simulink model "cte1"  (R2024b)
settings: Solver=ode15s  StartTime=0.0  StopTime=10.0  MaxStep=0.001  RelTol=1e-5
libraries: fl_lib x14, nesl_utility x6
settings Model: Creator=Apeksha  LastModifiedBy=hp

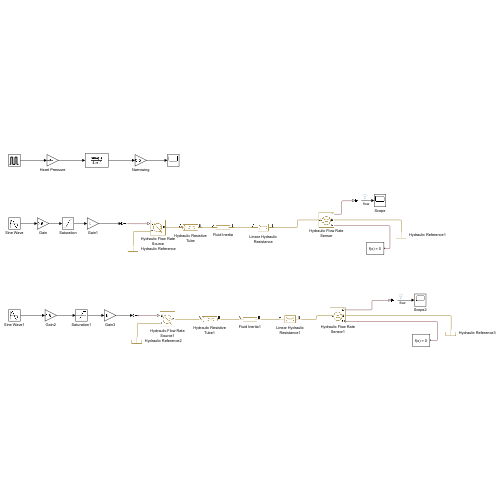
[thumbnail: Simulink's stored preview of the top-level diagram]
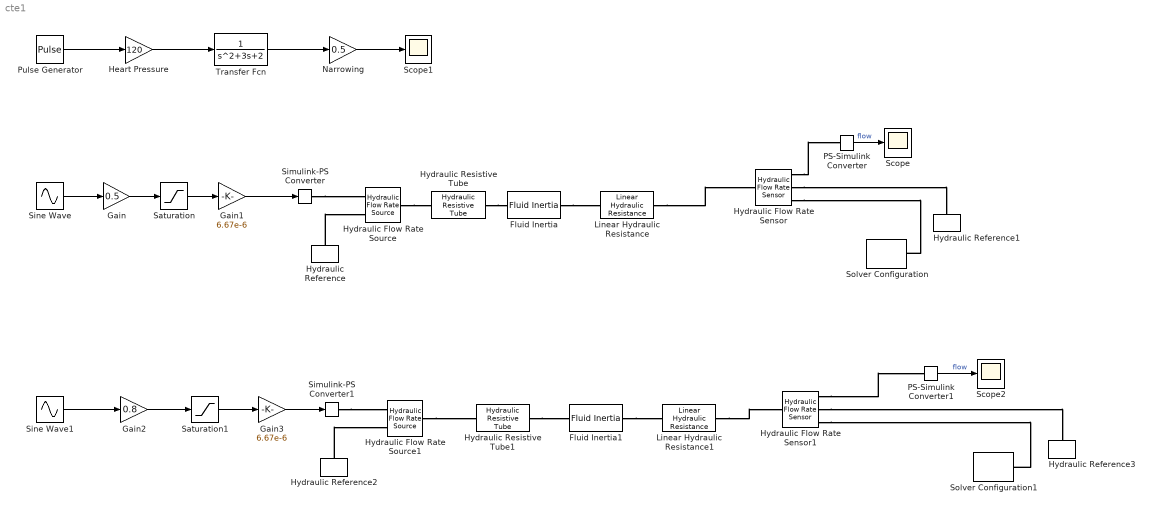
== system cte1 ==
  Fluid Inertia : fl_lib/Hydraulic/Hydraulic Elements/Fluid Inertia  area=0.8e-4 m^2  length=1 m  q_specify=on  q_priority=High  q=0 m^3/s  q_nominal_specify=off  q_nominal_value=1  q_nominal_unit=m^3/s  p_specify=on  p_priority=None  p=0 Pa  p_nominal_specify=off  p_nominal_value=1  p_nominal_unit=Pa
      settings: InternalSimscapePortConfiguration="{\"Bottom\":[],\"Left\":[{\"id\":\"A\",\"label\":\"A\",\"type\":\"foundation.hydraulic.hydraulic\"}],\"Right\":[{\"id\":\"B\",\"label\":\"B\",\"type\":\"foundation.hydraulic.hydraulic\"}],\"Top\":[]}"
  Fluid Inertia1 : fl_lib/Hydraulic/Hydraulic Elements/Fluid Inertia  area=0.8e-4 m^2  length=1 m  q_specify=on  q_priority=High  q=0 m^3/s  q_nominal_specify=off  q_nominal_value=1  q_nominal_unit=m^3/s  p_specify=on  p_priority=None  p=0 Pa  p_nominal_specify=off  p_nominal_value=1  p_nominal_unit=Pa
      settings: InternalSimscapePortConfiguration="{\"Bottom\":[],\"Left\":[{\"id\":\"A\",\"label\":\"A\",\"type\":\"foundation.hydraulic.hydraulic\"}],\"Right\":[{\"id\":\"B\",\"label\":\"B\",\"type\":\"foundation.hydraulic.hydraulic\"}],\"Top\":[]}"
  Gain : Gain  Gain=0.5
  Gain1 : Gain  Gain=6.67e-6
  Gain2 : Gain  Gain=0.8
  Gain3 : Gain  Gain=6.67e-6
  Heart Pressure : Gain  Gain=120
  Hydraulic Flow Rate Sensor : fl_lib/Hydraulic/Hydraulic Sensors/Hydraulic Flow Rate Sensor
  Hydraulic Flow Rate Sensor1 : fl_lib/Hydraulic/Hydraulic Sensors/Hydraulic Flow Rate Sensor
  Hydraulic Flow Rate Source : fl_lib/Hydraulic/Hydraulic Sources/Hydraulic Flow Rate Source
      settings: InternalSimscapePortConfiguration="{\"Bottom\":[],\"Left\":[{\"id\":\"P\",\"label\":\"P\",\"type\":\"foundation.hydraulic.hydraulic\"}],\"Right\":[{\"id\":\"S\",\"label\":\"S\",\"type\":\"input\"},{\"id\":\"T\",\"label\":\"T\",\"type\":\"foundation.hydraulic.hydraulic\"}],\"Top\":[]}"
  Hydraulic Flow Rate Source1 : fl_lib/Hydraulic/Hydraulic Sources/Hydraulic Flow Rate Source
      settings: InternalSimscapePortConfiguration="{\"Bottom\":[],\"Left\":[{\"id\":\"P\",\"label\":\"P\",\"type\":\"foundation.hydraulic.hydraulic\"}],\"Right\":[{\"id\":\"S\",\"label\":\"S\",\"type\":\"input\"},{\"id\":\"T\",\"label\":\"T\",\"type\":\"foundation.hydraulic.hydraulic\"}],\"Top\":[]}"
  Hydraulic Reference{,1..3} (4 alike) : fl_lib/Hydraulic/Hydraulic Elements/Hydraulic Reference
  Hydraulic Resistive Tube : fl_lib/Hydraulic/Hydraulic Elements/Hydraulic Resistive Tube  cs_type=1  d_in=0.01 m  area=1e-4 m^2  D_h=1.12e-2 m  s_factor=64  length=5 m  length_ad=1 m  roughness=15e-6 m  Re_lam=2000  Re_turb=4000  q_specify=off  q_priority=None  q=1e-3 m^3/s  q_nominal_specify=off  q_nominal_value=1  q_nominal_unit=m^3/s  p_specify=off  p_priority=None  p=0 Pa  p_nominal_specify=off  p_nominal_value=1  p_nominal_unit=Pa
      settings: InternalSimscapePortConfiguration="{\"Bottom\":[],\"Left\":[{\"id\":\"A\",\"label\":\"A\",\"type\":\"foundation.hydraulic.hydraulic\"}],\"Right\":[{\"id\":\"B\",\"label\":\"B\",\"type\":\"foundation.hydraulic.hydraulic\"}],\"Top\":[]}"
  Hydraulic Resistive Tube1 : fl_lib/Hydraulic/Hydraulic Elements/Hydraulic Resistive Tube  cs_type=1  d_in=0.01 m  area=1e-4 m^2  D_h=1.12e-2 m  s_factor=64  length=5 m  length_ad=1 m  roughness=15e-6 m  Re_lam=2000  Re_turb=4000  q_specify=off  q_priority=None  q=1e-3 m^3/s  q_nominal_specify=off  q_nominal_value=1  q_nominal_unit=m^3/s  p_specify=off  p_priority=None  p=0 Pa  p_nominal_specify=off  p_nominal_value=1  p_nominal_unit=Pa
      settings: InternalSimscapePortConfiguration="{\"Bottom\":[],\"Left\":[{\"id\":\"A\",\"label\":\"A\",\"type\":\"foundation.hydraulic.hydraulic\"}],\"Right\":[{\"id\":\"B\",\"label\":\"B\",\"type\":\"foundation.hydraulic.hydraulic\"}],\"Top\":[]}"
  Linear Hydraulic Resistance : fl_lib/Hydraulic/Hydraulic Elements/Linear Hydraulic Resistance  resistance=2.3e9 Pa*s/m^3  q_specify=on  q_priority=None  q=0 m^3/s  q_nominal_specify=on  q_nominal_value=3.33e-6  q_nominal_unit=m^3/s  p_specify=on  p_priority=None  p=0 Pa  p_nominal_specify=on  p_nominal_value=1.07e4  p_nominal_unit=Pa
      settings: InternalSimscapePortConfiguration="{\"Bottom\":[],\"Left\":[{\"id\":\"A\",\"label\":\"A\",\"type\":\"foundation.hydraulic.hydraulic\"}],\"Right\":[{\"id\":\"B\",\"label\":\"B\",\"type\":\"foundation.hydraulic.hydraulic\"}],\"Top\":[]}"
  Linear Hydraulic Resistance1 : fl_lib/Hydraulic/Hydraulic Elements/Linear Hydraulic Resistance  resistance=9.0e6 Pa*s/m^3  q_specify=on  q_priority=None  q=0 m^3/s  q_nominal_specify=on  q_nominal_value=3.33e-6  q_nominal_unit=m^3/s  p_specify=on  p_priority=None  p=0 Pa  p_nominal_specify=on  p_nominal_value=1.07e4  p_nominal_unit=Pa
      settings: InternalSimscapePortConfiguration="{\"Bottom\":[],\"Left\":[{\"id\":\"A\",\"label\":\"A\",\"type\":\"foundation.hydraulic.hydraulic\"}],\"Right\":[{\"id\":\"B\",\"label\":\"B\",\"type\":\"foundation.hydraulic.hydraulic\"}],\"Top\":[]}"
  Narrowing : Gain  Gain=0.5
  PS-Simulink Converter : nesl_utility/PS-Simulink Converter  PhysicalDomain=network_engine_domain  SubClassName=ps_output  LeftPortType=input  RightPortType=output  PseudoPeriodic=off  Frequencies=[]  VectorFormat=inherit  Unit=inherit  AffineConversion=off
  PS-Simulink Converter1 : nesl_utility/PS-Simulink Converter  PhysicalDomain=network_engine_domain  SubClassName=ps_output  LeftPortType=input  RightPortType=output  PseudoPeriodic=off  Frequencies=[]  VectorFormat=inherit  Unit=inherit  AffineConversion=off
  Pulse Generator : DiscretePulseGenerator  PulseType=Time based  Period=1  PulseWidth=5
  Saturation : Saturate  UpperLimit=1  LowerLimit=0
  Saturation1 : Saturate  UpperLimit=1  LowerLimit=0
  Scope : Scope
  Scope1 : Scope
  Scope2 : Scope
  Simulink-PS Converter : nesl_utility/Simulink-PS Converter  PhysicalDomain=network_engine_domain  SubClassName=ps_input  LeftPortType=input  RightPortType=output  PseudoPeriodic=off  Frequencies=[]  NoiseDistribution=none  NoiseParameters=[]  Unit=1  AffineConversion=off  FilteringAndDerivatives=filter  SimscapeFilterOrder=1  InputFilterTimeConstant=0.01  UdotUserProvided=0
  Simulink-PS Converter1 : nesl_utility/Simulink-PS Converter  PhysicalDomain=network_engine_domain  SubClassName=ps_input  LeftPortType=input  RightPortType=output  PseudoPeriodic=off  Frequencies=[]  NoiseDistribution=none  NoiseParameters=[]  Unit=1  AffineConversion=off  FilteringAndDerivatives=filter  SimscapeFilterOrder=1  InputFilterTimeConstant=0.01  UdotUserProvided=0
  Sine Wave : Sin  Frequency=2*pi*1.2  SampleTime=0
  Sine Wave1 : Sin  Frequency=2*pi*1.2  SampleTime=0
  Solver Configuration : nesl_utility/Solver Configuration  PhysicalDomain=network_engine_domain  SubClassName=solver  LeftPortType=input  RightPortType=generic  Tones=[]  Harmonics=[]  SimulateNoise=off  Profile=off  UseLocalSampling=off  EnableSwitchedLinearOptims=on  FrequencyDomain=off  UseCCode=off  RelTol=0.001  AbsTol=0.001  MinStep=1e-09  ToWorkspace=off  RevertToSquareIcSolve=off  NumHomotopyIterations=100  PhasorMode=off  PhasorModeNumHarmonics=1  ConsistencySolver=NEWTON_XTOL_AFTER_FTOL  IndexReductionMethod=DerivativeReplacement  DoDC=off  ResidualTolerance=1e-09  ConsistencyTolSource=GLOBAL  ConsistencyAbsTol=0.001  ConsistencyRelTol=0.001  ConsistencyTolFactor=0.001  UseLocalSolver=off  LocalSolverChoice=NE_BACKWARD_EULER_ADVANCER  ResolveIndetEquations=on  FunctionEvalNumThread=1  LocalSolverSampleTime=0.001  DoFixedCost=off  MaxNonlinIter=3  MaxModeIter=2  ComputeImpulses=off  ImpulseIterations=2  LinearAlgebra=auto  LinearAlgebraNumThread=0  EquationFormulation=NE_TIME_EF  DelaysMemoryBudget=1024  AutomaticFiltering=on  FilteringTimeConstant=0.001  PartitionStorageMethod=AS_NEEDED  PartitionMemoryBudget=1024  PartitionMethod=ROBUST  MultibodyUseLocalSolver=off  MultibodyLocalSolverChoice=ODE1  MultibodyLocalSolverSampleTime=0.001
  Solver Configuration1 : nesl_utility/Solver Configuration  PhysicalDomain=network_engine_domain  SubClassName=solver  LeftPortType=input  RightPortType=generic  Tones=[]  Harmonics=[]  SimulateNoise=off  Profile=off  UseLocalSampling=off  EnableSwitchedLinearOptims=on  FrequencyDomain=off  UseCCode=off  RelTol=0.001  AbsTol=0.001  MinStep=1e-09  ToWorkspace=off  RevertToSquareIcSolve=off  NumHomotopyIterations=100  PhasorMode=off  PhasorModeNumHarmonics=1  ConsistencySolver=NEWTON_XTOL_AFTER_FTOL  IndexReductionMethod=DerivativeReplacement  DoDC=off  ResidualTolerance=1e-09  ConsistencyTolSource=GLOBAL  ConsistencyAbsTol=0.001  ConsistencyRelTol=0.001  ConsistencyTolFactor=0.001  UseLocalSolver=off  LocalSolverChoice=NE_BACKWARD_EULER_ADVANCER  ResolveIndetEquations=on  FunctionEvalNumThread=1  LocalSolverSampleTime=0.001  DoFixedCost=off  MaxNonlinIter=3  MaxModeIter=2  ComputeImpulses=off  ImpulseIterations=2  LinearAlgebra=auto  LinearAlgebraNumThread=0  EquationFormulation=NE_TIME_EF  DelaysMemoryBudget=1024  AutomaticFiltering=on  FilteringTimeConstant=0.001  PartitionStorageMethod=AS_NEEDED  PartitionMemoryBudget=1024  PartitionMethod=ROBUST  MultibodyUseLocalSolver=off  MultibodyLocalSolverChoice=ODE1  MultibodyLocalSolverSampleTime=0.001
  Transfer Fcn : TransferFcn  Denominator=[1 3 2]
  wires:
  PS-Simulink Converter/1 -> Scope/1  "flow"
  Sine Wave/1 -> Gain/1
  Gain/1 -> Saturation/1
  Saturation/1 -> Gain1/1
  Gain1/1 -> Simulink-PS Converter/1
  Gain2/1 -> Saturation1/1
  Saturation1/1 -> Gain3/1
  Sine Wave1/1 -> Gain2/1
  Gain3/1 -> Simulink-PS Converter1/1
  PS-Simulink Converter1/1 -> Scope2/1  "flow"
  Narrowing/1 -> Scope1/1
  Heart Pressure/1 -> Transfer Fcn/1
  Pulse Generator/1 -> Heart Pressure/1
  Transfer Fcn/1 -> Narrowing/1
  connections:
  Hydraulic Resistive Tube/RConn1 -- Fluid Inertia/LConn1
  Fluid Inertia/RConn1 -- Linear Hydraulic Resistance/LConn1
  Linear Hydraulic Resistance/RConn1 -- Hydraulic Flow Rate Sensor/LConn1
  Hydraulic Flow Rate Sensor/RConn1 -- PS-Simulink Converter/LConn1
  Hydraulic Flow Rate Source/LConn1 -- Hydraulic Resistive Tube/LConn1
  Simulink-PS Converter/RConn1 -- Hydraulic Flow Rate Source/RConn1
  Hydraulic Reference/LConn1 -- Hydraulic Flow Rate Source/RConn2
  Hydraulic Flow Rate Sensor/RConn3 -- Solver Configuration/RConn1
  Hydraulic Flow Rate Sensor/RConn2 -- Hydraulic Reference1/LConn1
  Hydraulic Flow Rate Sensor1/RConn2 -- Hydraulic Reference3/LConn1
  Hydraulic Reference2/LConn1 -- Hydraulic Flow Rate Source1/RConn2
  Linear Hydraulic Resistance1/RConn1 -- Hydraulic Flow Rate Sensor1/LConn1
  Hydraulic Flow Rate Source1/LConn1 -- Hydraulic Resistive Tube1/LConn1
  Hydraulic Flow Rate Sensor1/RConn3 -- Solver Configuration1/RConn1
  Fluid Inertia1/RConn1 -- Linear Hydraulic Resistance1/LConn1
  Hydraulic Resistive Tube1/RConn1 -- Fluid Inertia1/LConn1
  Simulink-PS Converter1/RConn1 -- Hydraulic Flow Rate Source1/RConn1
  Hydraulic Flow Rate Sensor1/RConn1 -- PS-Simulink Converter1/LConn1
